simulink model "SOCestimation2_1"  (R2016a)
settings: Solver=FixedStepAuto  StartTime=0.0  StopTime=2591940  FixedStep=60  RelTol=1e-3
values from neighbouring files (symbols this model uses):
  Ap = 2    [SOCestimation.m]
  c = [c b]    [SOCestimation.m]    (also in rfmatrix.m = get(h(i),'XData'))
  Ca1 = 1/(w_zarc1*0.67^2*Ra1)    [SOCestimation.m]
  Ca2 = 1/(w_zarc2*0.804^2*Ra2)    [SOCestimation.m]
  CAh = CAh0 - CAh0*(1/100)*(C_cal_sum+C_cyc_sum)    (= 78)    [SOCestimation.m]
  Cb1 = 1/(w_zarc1*10.886*Rb1)    [SOCestimation.m]
  Cb2 = 1/(w_zarc2*4.675*Rb2)    [SOCestimation.m]
  Cc1 = 1/(w_zarc1*Rc1)    [SOCestimation.m]
  Cc2 = 1/(w_zarc1*Rc2)    [SOCestimation.m]
  Cd1 = 1/(w_zarc1*(1/10.886)*Rd1)    [SOCestimation.m]
  Cd2 = 1/(w_zarc2*(1/4.675)*Rd2)    [SOCestimation.m]
  Ce1 = 1/(w_zarc1*(1/0.67^2)*Re1)    [SOCestimation.m]
  Ce2 = 1/(w_zarc2*(1/0.804^2)*Re2)    [SOCestimation.m]
  Cp = 73.2    [SOCestimation.m]
  Ef = 0.17    [SOCestimation.m]
  Ls = 1.9*10^(-8)    (= 1.9e-08)    [SOCestimation.m]
  mission_month_Irrad = Irradiance((1+(i-1)*43200):(43200*i))    [SOCestimation.m]
  N = 1    [SOCestimation.m]
  Np = ceil(NT/Ns)    [Prototype_Sizing.m]    (also in SOCestimation.m = 85)
  Npb = 6    [SOCestimation.m]
  Ns = floor(Vdc/((Vb_soc_max)))    [Prototype_Sizing.m]    (also in SOCestimation.m = 30)
  Nsb = 10    [SOCestimation.m]
  OCV = 27.*OCV    [SOCestimation.m]
  Pbess = 580.84e3    (= 580840)    [SOCestimation.m]
  Ra1 = (R1-Rc1-Rb1-Rd1)/2    [SOCestimation.m]
  Ra2 = (R2-Rc2-Rb2-Rd2)/2    [SOCestimation.m]
  Rb1 = 0.670*(R1-Rc1)/2    [SOCestimation.m]
  Rb2 = 0.804*(R2-Rc2)/2    [SOCestimation.m]
  Rc1 = 0.906*R1*(sin(0.5*pi*0.5/2))/(1+cos(0.5*pi*0.5/2))    [SOCestimation.m]
  Rc2 = 0.833*R2*(sin(0.8*pi*0.5/2))/(1+cos(0.8*pi*0.5/2))    [SOCestimation.m]
  Rd1 = 0.670*(R1-Rc1)/2    [SOCestimation.m]
  Rd2 = 0.804*(R2-Rc2)/2    [SOCestimation.m]
  Re1 = (R1-Rc1-Rb1-Rd1)/2    [SOCestimation.m]
  Re2 = (R2-Rc2-Rb2-Rd2)/2    [SOCestimation.m]
  Rin = 3.273    [SOCestimation.m]
  Rout = 9.12    [SOCestimation.m]
  Rs = Rs + Rs_i    [SOCestimation.m]
  SOC = [0    0.0500    0.1000    0.1500    0.2000    0.2500    0.3000    0.3500    0.4000    0.4500    0.5000    0.5500 0.6000    0.6500    0.7000    0.7500    0.8000    0.8500    0.9000    0.9500    1.0000]    [SOCestimation.m]
  SOCmax = 90    [SOCestimation.m]
  SOCmin = 10    [SOCestimation.m]
  Temp = 25+273.15    (= 298.15)    [SOCestimation.m]
  time = [pos_loc neg_loc]    [LF_SBAI.m]    (also in Lifetime_Degradation.m; Plot_Capacity.m = time/30; SOCestimation.m = time'; battery_lifetime.m)
  Uac = 440    [SOCestimation.m]
undefined symbols (not defined in the file or in its folder): i
libraries: powerlib x33, simulink x5
settings Model: Creator=GESEP  LastModifiedBy=T.i
settings GRTTargetCC: GeneratePreprocessorConditionals=Use local settings

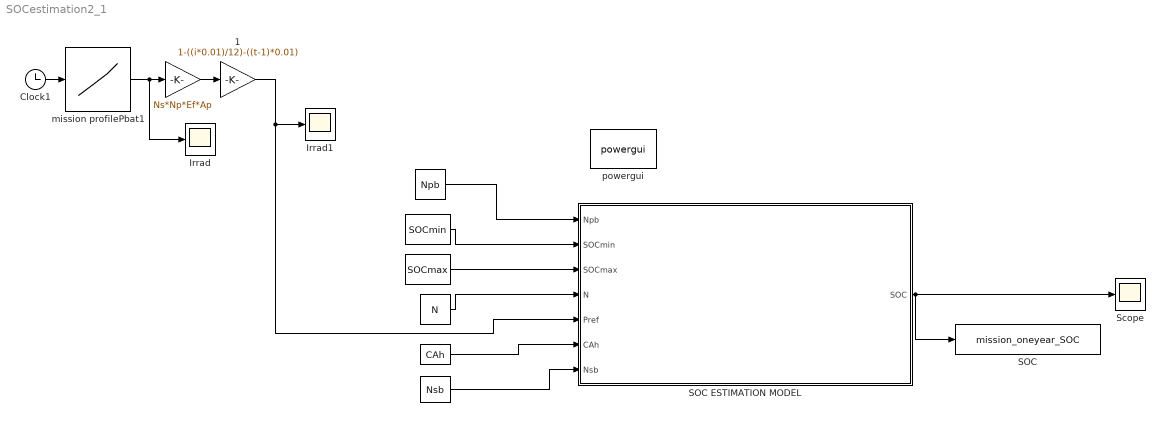
== system SOCestimation2_1 ==
  " " : Constant  Value=Nsb
  "  " : Constant  Value=Npb
  "    " : Constant  Value=SOCmin
  "        " : Constant  Value=SOCmax
  " " : Constant  Value=CAh
  "            " : Gain  Gain=Ns*Np*Ef*Ap
  "                " : Constant  Value=N
  "            1" : Gain  Gain=1-((i*0.01)/12)-((t-1)*0.01)
  Clock1 : Clock
  Irrad : Scope
  Irrad1 : Scope
  SOC : ToWorkspace  VariableName=mission_oneyear_SOC  SampleTime=-1
  SOC ESTIMATION MODEL : Subsystem
  Scope : Scope
  mission profilePbat1 : Lookup_n-D  NumberOfTableDimensions=1  BreakpointsForDimension1=time  Table=mission_month_Irrad  ExtrapMethod=Clip  UseLastTableValue=on  RndMeth=Simplest  InputSameDT=on
  powergui : powerlib/powergui  Priority=1  SimulationMode=Discrete  SolverType=Tustin/Backward Euler (TBE)  SampleTime=60  frequency=60  SPID=off  DisableSnubberDevices=off  DisableRonSwitches=off  DisableVfSwitches=off  SwTol=0  DisplayEquations=off  Interpol=off  ExternalGateDelay=off  methode=off  Ts=10  FunctionMessages=off  echomessages=off  HookPort=off  EnableUseOfTLC=off  x0status=blocks  frequencyindice=0  Pbase=100e6  ErrMax=1e-4  Iterations=50  UnitsV=kV  UnitsW=MW  buscounter=0  RestoreLinks=warning  ResistiveCurrentMeasurement=off  Frange=[0:2:500]  Ylog=off  Xlog=on  ShowGrid=off  save=off  variable=ZData  structure=0  ZoomFFT=off  StartTime=0.0  cycles=1  DisplayStyle=1  fundamental=60  FreqAxis=off  MaxFrequency=1000  frequencyindicesteady=1  RmsSteady=1  display=off
  wires:
  "  "/1 -> SOC ESTIMATION MODEL/1(Npb)
  " "/1 -> SOC ESTIMATION MODEL/7("Nsb ")
  "    "/1 -> SOC ESTIMATION MODEL/2(SOCmin)
  "        "/1 -> SOC ESTIMATION MODEL/3(SOCmax)
  "                "/1 -> SOC ESTIMATION MODEL/4(N)
  SOC ESTIMATION MODEL/1(SOC) -> SOC/1, Scope/1
  " "/1 -> SOC ESTIMATION MODEL/6(CAh)
  "            "/1 -> "            1"/1
  mission profilePbat1/1 -> Irrad/1, "            "/1
  Clock1/1 -> mission profilePbat1/1
  "            1"/1 -> SOC ESTIMATION MODEL/5(Pref), Irrad1/1

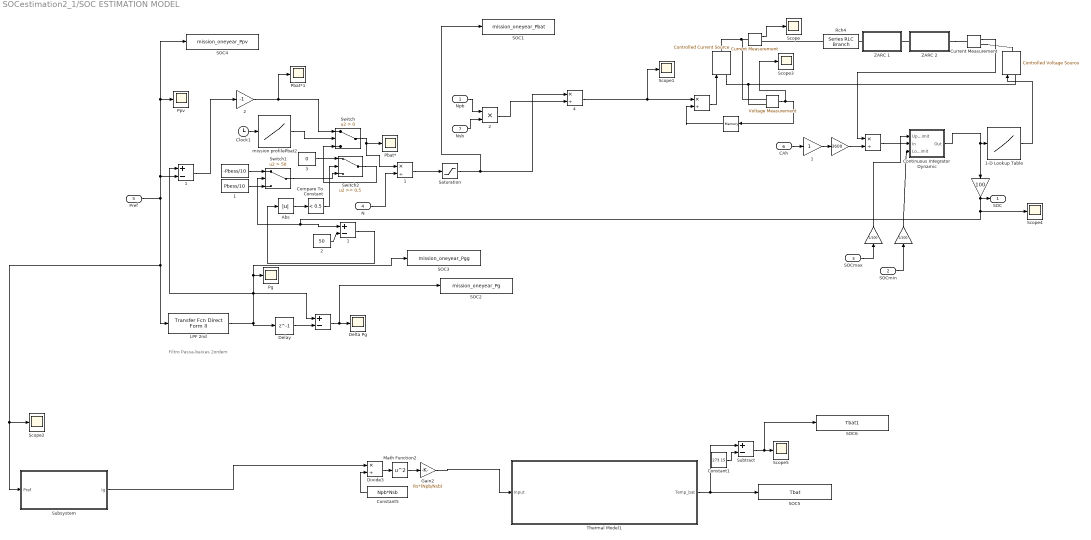
== system SOCestimation2_1/SOC ESTIMATION MODEL ==
  note: Filtro Passa-baixas 2ordem
  Npb : Inport
  SOCmin : Inport  Port=2
  SOCmax : Inport  Port=3
  N : Inport  Port=4
  Pref : Inport  Port=5
  CAh : Inport  Port=6
  "Nsb " : Inport  Port=7
  " " : Gain  Gain=3600
  "     " : Gain  Gain=100
  "      " : Gain  Gain=1/100
  "       " : Gain  Gain=1/100
  " " : Constant  Value=-Pbess/10
  " 1" : Constant  Value=Pbess/10
  " 2" : Constant  Value=50
  " 3" : Constant  Value=0
  "          " : powerlib/Measurements/Voltage Measurement  PhasorSimulation=off  OutputType=Complex  PSBequivalent=0
  "                 " : Memory  X0=2150
  "                      " : Sum  Inputs=+-
  "                            " : Product  Inputs=*/
  "                                   " : powerlib/Measurements/Current Measurement  PhasorSimulation=off  OutputType=Complex  PSBequivalent=0
  "                                           " : Product  Inputs=*/
  "                                                          " : powerlib/Electrical Sources/Controlled Voltage Source  Initialize=off  Source_Type=AC  Amplitude=20  Phase=2  Frequency=60  Measurements=None
  "                                                            " : powerlib/Electrical Sources/Controlled Current Source  Initialize=off  Source_Type=AC  Amplitude=20  Phase=2  Frequency=60  Measurements=None
  "                                           1" : Product  Inputs=*/
  "                                           2" : Product  Inputs=**
  "                                           4" : Product  Inputs=*/
  "                      1" : Sum  Inputs=+-
  "        1" : Sum  Inputs=+-
  " 1" : Gain
  " 2" : Gain  Gain=-1
  " Pg" : Scope
  1-D Lookup Table : Lookup_n-D  NumberOfTableDimensions=1  BreakpointsForDimension1=SOC  Table=OCV  InternalRulePriority=Speed  RndMeth=Simplest  InputSameDT=on
  Abs : Abs
  Clock1 : Clock
  Compare To Constant : simulink/Logic and Bit Operations/Compare To Constant  relop=<  const=0.5  OutDataTypeStr=boolean
  Constant1 : Constant  Value=273.15
  Constant5 : Constant  Value=Npb*Nsb
  Continuous Integrator Dynamic : Subsystem
  Current Measurement : powerlib/Measurements/Current Measurement  PhasorSimulation=off  OutputType=Complex  PSBequivalent=0
  Delay : Delay  DelayLength=1
  Delta Pg : Scope
  Divide3 : Product  Inputs=*/
  Gain2 : Gain  Gain=Rs*(Npb/Nsb)
  LPF 2nd : simulink/Additional Math & Discrete/Additional Discrete/Transfer Fcn Direct Form II  NumCoefVec=[0 0 (60/270)^2]  DenCoefVec=[(2*0.707*(1/270)*60 - 2) (1-2*0.707*(1/270)*60+60^2*(1/270)^2)]  vinit=0.0  DoSatur=off
  Math Function2 : Math  Operator=square  SaturateOnIntegerOverflow=on
  Pbat* : Scope
  Pbat*1 : Scope
  Ppv : Scope
  Rch4 : powerlib/Elements/Series RLC Branch  LConnTagsString=__new0  RConnTagsString=__new0  BranchType=R  Resistance=Rs  Inductance=1e-3  SetiL0=off  InitialCurrent=0  Capacitance=1e-6  Setx0=off  InitialVoltage=0  Measurements=None
  SOC1 : ToWorkspace  VariableName=mission_oneyear_Pbat  SampleTime=-1
  SOC2 : ToWorkspace  VariableName=mission_oneyear_Pg  SampleTime=-1
  SOC3 : ToWorkspace  VariableName=mission_oneyear_Pgg  SampleTime=-1
  SOC4 : ToWorkspace  VariableName=mission_oneyear_Ppv  SampleTime=-1
  SOC5 : ToWorkspace  VariableName=Tbat  SampleTime=-1
  SOC6 : ToWorkspace  VariableName=Tbat1  SampleTime=-1
  Saturation : Saturate  UpperLimit=Pbess  LowerLimit=-Pbess
  Scope{,1..5} (6 alike) : Scope
  Subsystem : Subsystem
  Subtract : Sum  Inputs=+-
  Switch : Switch  Criteria=u2 > Threshold
  Switch1 : Switch  Criteria=u2 > Threshold  Threshold=50
  Switch2 : Switch  Threshold=0.5
  Thermal Model1 : Subsystem
  ZARC 1 : Subsystem
  ZARC 2 : Subsystem
  mission profilePbat2 : Lookup_n-D  NumberOfTableDimensions=1  BreakpointsForDimension1=time  Table=c  ExtrapMethod=Clip  UseLastTableValue=on  RndMeth=Simplest  InputSameDT=on
  SOC : Outport
  wires:
  "                 "/1 -> "                                           "/2
  "                                           "/1 -> "                                                            "/1
  " "/1 -> "                            "/2
  Current Measurement/1 -> "                            "/1
  "          "/1 -> Scope3/1, "                 "/1
  SOCmax/1 -> "      "/1
  SOCmin/1 -> "       "/1
  "       "/1 -> Continuous Integrator Dynamic/3(Lower Limit)
  "      "/1 -> Continuous Integrator Dynamic/1(Upper Limit)
  "                                   "/1 -> Scope/1
  CAh/1 -> " 1"/1
  "                            "/1 -> Continuous Integrator Dynamic/2(In)
  1-D Lookup Table/1 -> "                                                          "/1
  Continuous Integrator Dynamic/1(Out) -> "     "/1, 1-D Lookup Table/1
  Clock1/1 -> mission profilePbat2/1
  " 3"/1 -> Switch2/1
  "     "/1 -> Scope4/1, Switch1/2, "                      1"/1, SOC/1
  " 2"/1 -> "                      1"/2
  mission profilePbat2/1 -> Switch/2
  "                      1"/1 -> Abs/1
  Switch/1 -> "                                           1"/1, Pbat*/1
  Switch1/1 -> Switch2/3
  N/1 -> "                                           1"/2
  Abs/1 -> Compare To Constant/1
  Compare To Constant/1 -> Switch2/2
  Switch2/1 -> Switch/3
  Delay/1 -> "                      "/2
  "                      "/1 -> SOC2/1, Delta Pg/1
  " "/1 -> Switch1/1
  " 1"/1 -> Switch1/3
  "        1"/1 -> " 2"/1
  LPF 2nd/1 -> SOC3/1, " Pg"/1, "                      "/1, "        1"/1, Delay/1
  " 1"/1 -> " "/1
  Npb/1 -> "                                           2"/1
  "Nsb "/1 -> "                                           2"/2
  "                                           2"/1 -> "                                           4"/2
  "                                           4"/1 -> Scope1/1, "                                           "/1
  " 2"/1 -> Pbat*1/1, Switch/1
  Gain2/1 -> Thermal Model1/1(Input)
  Thermal Model1/1("Temp_bat ") -> SOC5/1, Subtract/1
  Subsystem/1(Ig) -> Divide3/1
  Constant1/1 -> Subtract/2
  Constant5/1 -> Divide3/2
  Divide3/1 -> Math Function2/1
  Math Function2/1 -> Gain2/1
  Pref/1 -> "        1"/2, SOC4/1, Ppv/1, Scope2/1, Subsystem/1(Pref), LPF 2nd/1
  Subtract/1 -> SOC6/1, Scope5/1
  "                                           1"/1 -> Saturation/1
  Saturation/1 -> SOC1/1, "                                           4"/1
  connections:
  "                                                            "/LConn1 -- "                                                          "/LConn1 -- "          "/LConn2
  Current Measurement/RConn1 -- "                                                          "/RConn1
  "          "/LConn1 -- "                                   "/LConn1 -- "                                                            "/RConn1
  ZARC 2/RConn1 -- Current Measurement/LConn1
  ZARC 1/LConn1 -- Rch4/LConn1
  ZARC 2/LConn1 -- ZARC 1/RConn1
  Rch4/RConn1 -- "                                   "/RConn1

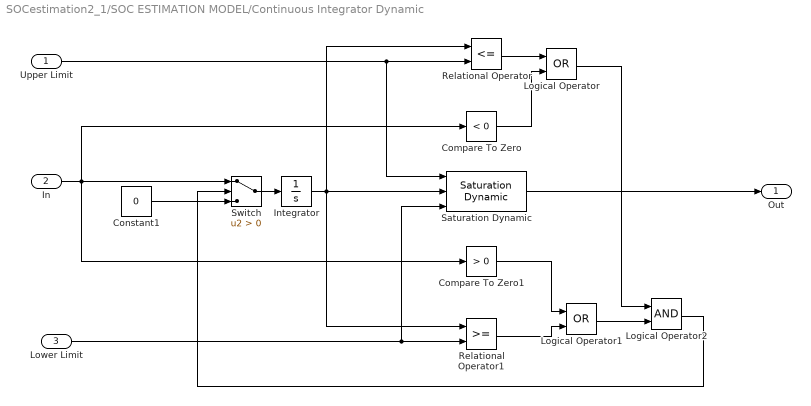
== system SOCestimation2_1/SOC ESTIMATION MODEL/Continuous Integrator Dynamic ==
  Upper Limit : Inport
  In : Inport  Port=2
  Lower Limit : Inport  Port=3
  Compare To Zero : simulink/Logic and Bit Operations/Compare To Zero  relop=<  OutDataTypeStr=uint8  ZeroCross=off
  Compare To Zero1 : simulink/Logic and Bit Operations/Compare To Zero  relop=>  OutDataTypeStr=uint8  ZeroCross=off
  Constant1 : Constant  Value=0
  Integrator : Integrator
  Logical Operator : Logic  Operator=OR  AllPortsSameDT=off  OutDataTypeStr=boolean
  Logical Operator1 : Logic  Operator=OR  AllPortsSameDT=off  OutDataTypeStr=boolean
  Logical Operator2 : Logic  AllPortsSameDT=off  OutDataTypeStr=boolean
  Relational Operator : RelationalOperator  Operator=<=  OutDataTypeStr=boolean
  Relational Operator1 : RelationalOperator  OutDataTypeStr=boolean
  Saturation Dynamic : simulink/Discontinuities/Saturation Dynamic  OutMin=[]  OutMax=[]  OutDataTypeStr=Inherit: Same as second input  OutDataType=fixdt(1, 16)  OutScaling=2^-10  DoSatur=off
  Switch : Switch  Criteria=u2 > Threshold
  Out : Outport
  wires:
  In/1 -> Compare To Zero/1, Compare To Zero1/1, Switch/1
  Constant1/1 -> Switch/3
  Switch/1 -> Integrator/1
  Relational Operator/1 -> Logical Operator/1
  Compare To Zero/1 -> Logical Operator/2
  Upper Limit/1 -> Relational Operator/2, Saturation Dynamic/1
  Lower Limit/1 -> Relational Operator1/2, Saturation Dynamic/3
  Compare To Zero1/1 -> Logical Operator1/1
  Relational Operator1/1 -> Logical Operator1/2
  Logical Operator1/1 -> Logical Operator2/2
  Logical Operator/1 -> Logical Operator2/1
  Logical Operator2/1 -> Switch/2
  Saturation Dynamic/1 -> Out/1
  Integrator/1 -> Relational Operator/1, Relational Operator1/1, Saturation Dynamic/2

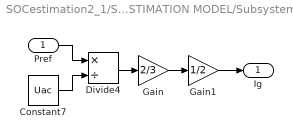
== system SOCestimation2_1/SOC ESTIMATION MODEL/Subsystem ==
  Pref : Inport
  Constant7 : Constant  Value=Uac
  Divide4 : Product  Inputs=*/
  Gain : Gain  Gain=2/3
  Gain1 : Gain  Gain=1/2
  Ig : Outport
  wires:
  Divide4/1 -> Gain/1
  Constant7/1 -> Divide4/2
  Pref/1 -> Divide4/1
  Gain/1 -> Gain1/1
  Gain1/1 -> Ig/1

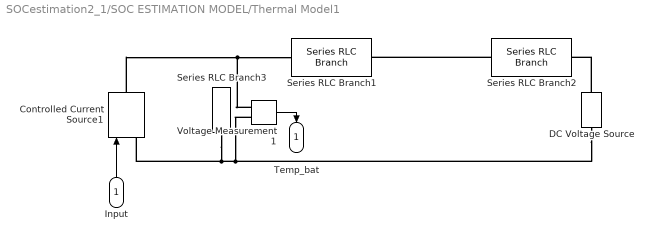
== system SOCestimation2_1/SOC ESTIMATION MODEL/Thermal Model1 ==
  Input : Inport
  Controlled Current Source1 : powerlib/Electrical Sources/Controlled Current Source  Initialize=off  Source_Type=DC  Amplitude=2150  Phase=0  Frequency=0  Measurements=None
  DC Voltage Source : powerlib/Electrical Sources/DC Voltage Source  Amplitude=Temp  Measurements=None
  Series RLC Branch1 : powerlib/Elements/Series RLC Branch  LConnTagsString=__new0  RConnTagsString=__new0  BranchType=R  Resistance=Rin  Inductance=Ls  SetiL0=off  InitialCurrent=2  Capacitance=1e-6  Setx0=off  InitialVoltage=0  Measurements=None
  Series RLC Branch2 : powerlib/Elements/Series RLC Branch  LConnTagsString=__new0  RConnTagsString=__new0  BranchType=R  Resistance=Rout  Inductance=Ls  SetiL0=off  InitialCurrent=2  Capacitance=1e-6  Setx0=off  InitialVoltage=0  Measurements=None
  Series RLC Branch3 : powerlib/Elements/Series RLC Branch  LConnTagsString=__new0  RConnTagsString=__new0  BranchType=C  Resistance=Rs  Inductance=Ls  SetiL0=off  InitialCurrent=2  Capacitance=Cp  Setx0=off  InitialVoltage=25+273.15  Measurements=None
  Voltage Measurement1 : powerlib/Measurements/Voltage Measurement  PhasorSimulation=off  OutputType=Complex  PSBequivalent=0
  "Temp_bat " : Outport
  wires:
  Input/1 -> Controlled Current Source1/1
  Voltage Measurement1/1 -> "Temp_bat "/1
  connections:
  DC Voltage Source/LConn1 -- Voltage Measurement1/LConn2 -- Series RLC Branch3/RConn1 -- Controlled Current Source1/LConn1
  Controlled Current Source1/RConn1 -- Voltage Measurement1/LConn1 -- Series RLC Branch1/LConn1
  Series RLC Branch2/LConn1 -- Series RLC Branch1/RConn1
  DC Voltage Source/RConn1 -- Series RLC Branch2/RConn1

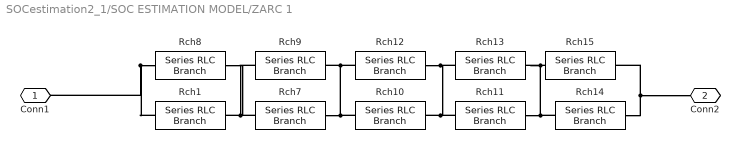
== system SOCestimation2_1/SOC ESTIMATION MODEL/ZARC 1 ==
  Rch1 : powerlib/Elements/Series RLC Branch  LConnTagsString=__new0  RConnTagsString=__new0  BranchType=R  Resistance=Ra1  Inductance=1e-3  SetiL0=off  InitialCurrent=0  Capacitance=1e-6  Setx0=off  InitialVoltage=0  Measurements=None
  Rch10 : powerlib/Elements/Series RLC Branch  LConnTagsString=__new0  RConnTagsString=__new0  BranchType=R  Resistance=Rc1  Inductance=1e-3  SetiL0=off  InitialCurrent=0  Capacitance=1e-6  Setx0=off  InitialVoltage=0  Measurements=None
  Rch11 : powerlib/Elements/Series RLC Branch  LConnTagsString=__new0  RConnTagsString=__new0  BranchType=R  Resistance=Rd1  Inductance=1e-3  SetiL0=off  InitialCurrent=0  Capacitance=1e-6  Setx0=off  InitialVoltage=0  Measurements=None
  Rch12 : powerlib/Elements/Series RLC Branch  LConnTagsString=__new0  RConnTagsString=__new0  BranchType=C  Resistance=0.01304  Inductance=1e-3  SetiL0=off  InitialCurrent=0  Capacitance=Cc1  Setx0=off  InitialVoltage=0  Measurements=None
  Rch13 : powerlib/Elements/Series RLC Branch  LConnTagsString=__new0  RConnTagsString=__new0  BranchType=C  Resistance=0.01304  Inductance=1e-3  SetiL0=off  InitialCurrent=0  Capacitance=Cd1  Setx0=off  InitialVoltage=0  Measurements=None
  Rch14 : powerlib/Elements/Series RLC Branch  LConnTagsString=__new0  RConnTagsString=__new0  BranchType=R  Resistance=Re1  Inductance=1e-3  SetiL0=off  InitialCurrent=0  Capacitance=1e-6  Setx0=off  InitialVoltage=0  Measurements=None
  Rch15 : powerlib/Elements/Series RLC Branch  LConnTagsString=__new0  RConnTagsString=__new0  BranchType=C  Resistance=0.01304  Inductance=1e-3  SetiL0=off  InitialCurrent=0  Capacitance=Ce1  Setx0=off  InitialVoltage=0  Measurements=None
  Rch7 : powerlib/Elements/Series RLC Branch  LConnTagsString=__new0  RConnTagsString=__new0  BranchType=R  Resistance=Rb1  Inductance=1e-3  SetiL0=off  InitialCurrent=0  Capacitance=1e-6  Setx0=off  InitialVoltage=0  Measurements=None
  Rch8 : powerlib/Elements/Series RLC Branch  LConnTagsString=__new0  RConnTagsString=__new0  BranchType=C  Resistance=0.01304  Inductance=1e-3  SetiL0=off  InitialCurrent=0  Capacitance=Ca1  Setx0=off  InitialVoltage=0  Measurements=None
  Rch9 : powerlib/Elements/Series RLC Branch  LConnTagsString=__new0  RConnTagsString=__new0  BranchType=C  Resistance=0.01304  Inductance=1e-3  SetiL0=off  InitialCurrent=0  Capacitance=Cb1  Setx0=off  InitialVoltage=0  Measurements=None
  Conn1 : PMIOPort  Port=1  Side=Left
  Conn2 : PMIOPort  Port=2  Side=Right
  connections:
  Rch14/LConn1 -- Conn2/RConn1 -- Rch15/LConn1
  Rch7/LConn1 -- Rch10/RConn1 -- Rch12/RConn1 -- Rch9/LConn1
  Rch8/RConn1 -- Conn1/RConn1 -- Rch1/RConn1
  Rch7/RConn1 -- Rch1/LConn1 -- Rch8/LConn1 -- Rch9/RConn1
  Rch11/LConn1 -- Rch14/RConn1 -- Rch15/RConn1 -- Rch13/LConn1
  Rch13/RConn1 -- Rch12/LConn1 -- Rch10/LConn1 -- Rch11/RConn1

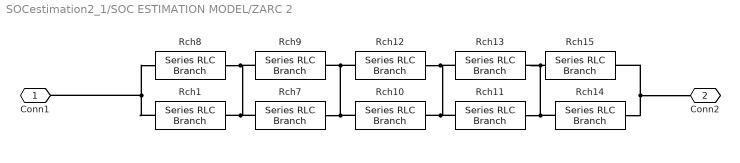
== system SOCestimation2_1/SOC ESTIMATION MODEL/ZARC 2 ==
  Rch1 : powerlib/Elements/Series RLC Branch  LConnTagsString=__new0  RConnTagsString=__new0  BranchType=R  Resistance=Ra2  Inductance=1e-3  SetiL0=off  InitialCurrent=0  Capacitance=1e-6  Setx0=off  InitialVoltage=0  Measurements=None
  Rch10 : powerlib/Elements/Series RLC Branch  LConnTagsString=__new0  RConnTagsString=__new0  BranchType=R  Resistance=Rc2  Inductance=1e-3  SetiL0=off  InitialCurrent=0  Capacitance=1e-6  Setx0=off  InitialVoltage=0  Measurements=None
  Rch11 : powerlib/Elements/Series RLC Branch  LConnTagsString=__new0  RConnTagsString=__new0  BranchType=R  Resistance=Rd2  Inductance=1e-3  SetiL0=off  InitialCurrent=0  Capacitance=1e-6  Setx0=off  InitialVoltage=0  Measurements=None
  Rch12 : powerlib/Elements/Series RLC Branch  LConnTagsString=__new0  RConnTagsString=__new0  BranchType=C  Resistance=0.01304  Inductance=1e-3  SetiL0=off  InitialCurrent=0  Capacitance=Cc2  Setx0=off  InitialVoltage=0  Measurements=None
  Rch13 : powerlib/Elements/Series RLC Branch  LConnTagsString=__new0  RConnTagsString=__new0  BranchType=C  Resistance=0.01304  Inductance=1e-3  SetiL0=off  InitialCurrent=0  Capacitance=Cd2  Setx0=off  InitialVoltage=0  Measurements=None
  Rch14 : powerlib/Elements/Series RLC Branch  LConnTagsString=__new0  RConnTagsString=__new0  BranchType=R  Resistance=Re2  Inductance=1e-3  SetiL0=off  InitialCurrent=0  Capacitance=1e-6  Setx0=off  InitialVoltage=0  Measurements=None
  Rch15 : powerlib/Elements/Series RLC Branch  LConnTagsString=__new0  RConnTagsString=__new0  BranchType=C  Resistance=0.01304  Inductance=1e-3  SetiL0=off  InitialCurrent=0  Capacitance=Ce2  Setx0=off  InitialVoltage=0  Measurements=None
  Rch7 : powerlib/Elements/Series RLC Branch  LConnTagsString=__new0  RConnTagsString=__new0  BranchType=R  Resistance=Rb2  Inductance=1e-3  SetiL0=off  InitialCurrent=0  Capacitance=1e-6  Setx0=off  InitialVoltage=0  Measurements=None
  Rch8 : powerlib/Elements/Series RLC Branch  LConnTagsString=__new0  RConnTagsString=__new0  BranchType=C  Resistance=0.01304  Inductance=1e-3  SetiL0=off  InitialCurrent=0  Capacitance=Ca2  Setx0=off  InitialVoltage=0  Measurements=None
  Rch9 : powerlib/Elements/Series RLC Branch  LConnTagsString=__new0  RConnTagsString=__new0  BranchType=C  Resistance=0.01304  Inductance=1e-3  SetiL0=off  InitialCurrent=0  Capacitance=Cb2  Setx0=off  InitialVoltage=0  Measurements=None
  Conn1 : PMIOPort  Port=1  Side=Left
  Conn2 : PMIOPort  Port=2  Side=Right
  connections:
  Rch15/LConn1 -- Rch14/LConn1 -- Conn2/RConn1
  Rch9/LConn1 -- Rch10/RConn1 -- Rch7/LConn1 -- Rch12/RConn1
  Rch1/RConn1 -- Rch8/RConn1 -- Conn1/RConn1
  Rch9/RConn1 -- Rch1/LConn1 -- Rch7/RConn1 -- Rch8/LConn1
  Rch15/RConn1 -- Rch13/LConn1 -- Rch11/LConn1 -- Rch14/RConn1
  Rch11/RConn1 -- Rch12/LConn1 -- Rch13/RConn1 -- Rch10/LConn1
